simulink model "controle_modelo"  (R2025a)
settings: Solver=VariableStepAuto  StartTime=0.0  StopTime=300.0  RelTol=1e-3
values from neighbouring files (symbols this model uses):
  alpha_p = 5    [controle_modelo_aloc.m]
  alpha_ti = 1    [controle_modelo_aloc.m]
  Kc1 = Kc1*(lambda - sqrt(lambda^2 - lambda))    [controle_modelo_aloc.m]
  Kc2 = Kc2*(lambda - sqrt(lambda^2 - lambda))    [controle_modelo_aloc.m]
  Ti1 = Kp1 / Ki1    (= 17.2152739347)    [controle_modelo_aloc.m]
  Ti2 = Kp2 / Ki2    (= 36.9239766082)    [controle_modelo_aloc.m]
libraries: cstblocks x4
settings Model: Creator=joaof  LastModifiedBy=joaof

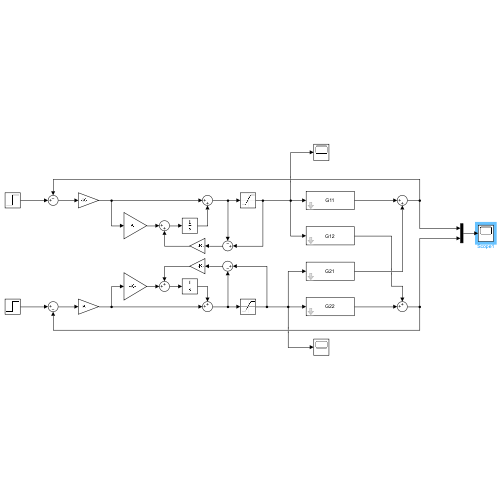
[thumbnail: Simulink's stored preview of the top-level diagram]
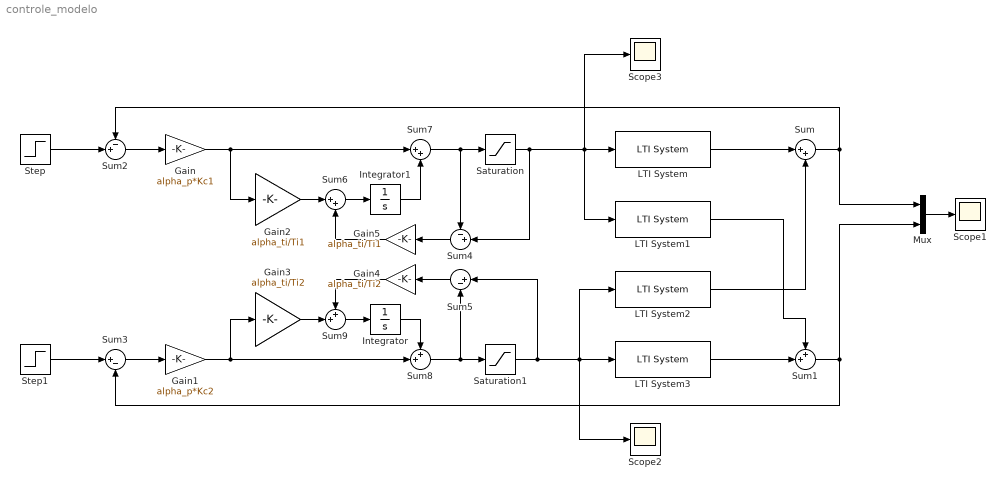
== system controle_modelo ==
  Gain : Gain  Gain=alpha_p*Kc1
  Gain1 : Gain  Gain=alpha_p*Kc2
  Gain2 : Gain  Gain=alpha_ti/Ti1
  Gain3 : Gain  Gain=alpha_ti/Ti2
  Gain4 : Gain  Gain=alpha_ti/Ti2
  Gain5 : Gain  Gain=alpha_ti/Ti1
  Integrator : Integrator
  Integrator1 : Integrator
  LTI System : cstblocks/LTI System  sys=G11  IC=[]  PadeOrder=0
  LTI System1 : cstblocks/LTI System  sys=G12  IC=[]  PadeOrder=0
  LTI System2 : cstblocks/LTI System  sys=G21  IC=[]  PadeOrder=0
  LTI System3 : cstblocks/LTI System  sys=G22  IC=[]  PadeOrder=0
  Mux : Mux  Inputs=2
  Saturation : Saturate  UpperLimit=10  LowerLimit=0
  Saturation1 : Saturate  UpperLimit=10  LowerLimit=0
  Scope1 : Scope
      settings: ActiveDisplayYMinimum=-0.049414403031056896  ActiveDisplayYMaximum=0.44472962727951221
  Scope2 : Scope
      settings: ActiveDisplayYMinimum=-1.2499999999999998  ActiveDisplayYMaximum=11.25  DataLoggingVariableName=ScopeData2
  Scope3 : Scope
      settings: ActiveDisplayYMinimum=-1.2499999999999998  ActiveDisplayYMaximum=11.25  DataLoggingVariableName=ScopeData3
  Step : Step  Before=0.25  After=0.28  SampleTime=0
  Step1 : Step  Before=0.35  After=0.38  SampleTime=0
  Sum : Sum  Inputs=|++
  Sum1 : Sum  Inputs=++|
  Sum2 : Sum  Inputs=-+|
  Sum3 : Sum  Inputs=|+-
  Sum4 : Sum  Inputs=-+|
  Sum5 : Sum  Inputs=|+-
  Sum6 : Sum  Inputs=|++
  Sum7 : Sum  Inputs=|++
  Sum8 : Sum  Inputs=++|
  Sum9 : Sum  Inputs=++|
  wires:
  LTI System3/1 -> Sum1/2
  LTI System/1 -> Sum/1
  Sum/1 -> Mux/1, Sum2/1
  LTI System2/1 -> Sum/2
  LTI System1/1 -> Sum1/1
  Sum1/1 -> Mux/2, Sum3/2
  Gain/1 -> Gain2/1, Sum7/1
  Sum2/1 -> Gain/1
  Sum8/1 -> Sum5/2, Saturation1/1
  Step/1 -> Sum2/2
  Step1/1 -> Sum3/1
  Saturation/1 -> Sum4/2, Scope3/1, LTI System1/1, LTI System/1
  Saturation1/1 -> Sum5/1, Scope2/1, LTI System2/1, LTI System3/1
  Gain2/1 -> Sum6/1
  Sum4/1 -> Gain5/1
  Sum7/1 -> Sum4/1, Saturation/1
  Sum3/1 -> Gain1/1
  Gain1/1 -> Gain3/1, Sum8/2
  Gain3/1 -> Sum9/2
  Sum5/1 -> Gain4/1
  Sum9/1 -> Integrator/1
  Integrator/1 -> Sum8/1
  Sum6/1 -> Integrator1/1
  Integrator1/1 -> Sum7/2
  Gain4/1 -> Sum9/1
  Gain5/1 -> Sum6/2
  Mux/1 -> Scope1/1
